simulink model "BESS_F_V_Controle"  (R2017b)
settings: Solver=ode45  StartTime=0.0  StopTime=10  RelTol=1e-3  EnableMultiTasking=on
values from neighbouring files (symbols this model uses):
  beta = beta (k)    [Parameter_2M_DFIG_BESS.m]
  Cbus = 80e-3    (= 0.08)    [Parameter_2M_DFIG_BESS.m]
  Cbus_bess = 15e-3    (= 0.015)    [Parameter_2M_DFIG_BESS.m]
  Cfilter = 80e-3    (= 0.08)    [Parameter_2M_DFIG_BESS.m]
  cp_opt_abs = abs(max(Cp))    [Parameter_2M_DFIG_BESS.m]
  D = 0.1    [Parameter_2M_DFIG_BESS.m]
  f = 60    [Parameter_2M_DFIG_BESS.m]
  Fs = 1.8    [Parameter_2M_DFIG_BESS.m]
  fsw = 4e3    (= 4000)    [Parameter_2M_DFIG_BESS.m]
  J = 90    [Parameter_2M_DFIG_BESS.m]
  ki_id = (wni^2)*Lr*sigma    (= 491.599501999)    [Parameter_2M_DFIG_BESS.m]
  ki_idg = (wnig^2)*Lg    (= 68.6450725305)    [Parameter_2M_DFIG_BESS.m]
  ki_iq = ki_id    (= 491.599501999)    [Parameter_2M_DFIG_BESS.m]
  ki_iqg = ki_idg    (= 68.6450725305)    [Parameter_2M_DFIG_BESS.m]
  ki_v = -300000    [Parameter_2M_DFIG_BESS.m]
  kp_id = (2*wni*sigma*Lr)-Rr    (= 0.5771)    [Parameter_2M_DFIG_BESS.m]
  kp_idg = (2*wnig*Lg)-Rg    (= 0.364153420404)    [Parameter_2M_DFIG_BESS.m]
  kp_iq = kp_id    (= 0.5771)    [Parameter_2M_DFIG_BESS.m]
  kp_iqg = kp_idg    (= 0.364153420404)    [Parameter_2M_DFIG_BESS.m]
  kp_v = -1000    [Parameter_2M_DFIG_BESS.m]
  Kpg = 1/(1.5*Vs*sqrt(2/3))    [Parameter_2M_DFIG_BESS.m]
  Kqg = -Kpg    [Parameter_2M_DFIG_BESS.m]
  lambda_opt = abs(lambda(posicion))    [Parameter_2M_DFIG_BESS.m]
  Lfilter = 483e-6    (= 0.000483)    [Parameter_2M_DFIG_BESS.m]
  Lg = 483e-6    (= 0.000483)    [Parameter_2M_DFIG_BESS.m]
  Lm = 2.5e-3    (= 0.0025)    [Parameter_2M_DFIG_BESS.m]
  Lr = Lm + Lsr    (= 0.002587)    [Parameter_2M_DFIG_BESS.m]
  Ls = Lm + Lsi    (= 0.002587)    [Parameter_2M_DFIG_BESS.m]
  Lsi = 87e-6    (= 8.7e-05)    [Parameter_2M_DFIG_BESS.m]
  N = 100    [Parameter_2M_DFIG_BESS.m]
  p = 2    [Parameter_2M_DFIG_BESS.m]
  Ps = 2e6    (= 2000000)    [Parameter_2M_DFIG_BESS.m]
  Radio = 44    [Parameter_2M_DFIG_BESS.m]
  Rfilter = 20e-3    (= 0.02)    [Parameter_2M_DFIG_BESS.m]
  Rg = 20e-6    (= 2e-05)    [Parameter_2M_DFIG_BESS.m]
  ro = 1.225    [Parameter_2M_DFIG_BESS.m]
  Rr = 2.9e-3    (= 0.0029)    [Parameter_2M_DFIG_BESS.m]
  Rs = 2.6e-3    (= 0.0026)    [Parameter_2M_DFIG_BESS.m]
  sigma = 1- Lm^2/(Ls*Lr)    (= 0.0661284179513)    [Parameter_2M_DFIG_BESS.m]
  Ts = 1/fsw/f    (= 4.16666666667e-06)    [Parameter_2M_DFIG_BESS.m]
  Vbus_ref = 1200    [Parameter_2M_DFIG_BESS.m]
  Vs = 690    [Parameter_2M_DFIG_BESS.m]
undefined symbols (not defined in the file or in its folder): D1, D11, Delta, DiscIntNeverNeededParam, Ion, Lithium, sigbuilder_block
libraries: powerlib x72, powerlib_meascontrol x37, electricdrivelib x1, simulink x1, sps_avr x1
(part 3 of 3)

== system BESS_F_V_Controle/BESS 1.0 MW 690 V/Control System/PI Iq1 ==
  Q*_ref : Inport
  Q_means : Inport  Port=2
  Discrete-Time Integrator : DiscreteIntegrator  SampleTime=1/fsw  LimitOutput=on  UpperSaturationLimit=1e6  LowerSaturationLimit=-Vbus_ref/sqrt(3)  ICPrevOutput=DiscIntNeverNeededParam  ICPrevScaledInput=DiscIntNeverNeededParam
  Error : Display
  Gain : Gain  Gain=kp_iqg
  Gain1 : Gain  Gain=ki_iqg
  Mean : Display
  Mux : Mux  Inputs=3
  Ref : Display
  Sat : Display
  Sat 1 : Display
  Saturation : Saturate  UpperLimit=1e6  LowerLimit=-1e6
  Scope : Scope
  Sum : Sum  Inputs=|+-
  Sum1 : Sum  Inputs=|++
  "Q " : Outport
  wires:
  Sum1/1 -> Saturation/1
  Discrete-Time Integrator/1 -> Sat 1/1, Sum1/2
  Gain1/1 -> Discrete-Time Integrator/1
  Gain/1 -> Sum1/1
  Saturation/1 -> Sat/1, "Q "/1
  Q_means/1 -> Sum/2, Mean/1, Mux/2
  Q*_ref/1 -> Sum/1, Ref/1, Mux/1
  Sum/1 -> Mux/3, Error/1, Gain/1, Gain1/1
  Mux/1 -> Scope/1

== system BESS_F_V_Controle/BESS 1.0 MW 690 V/Control System/PI Iq3 ==
  Vq*_ref : Inport
  Vq_means : Inport  Port=2
  Discrete-Time Integrator : DiscreteIntegrator  SampleTime=1/fsw  LimitOutput=on  UpperSaturationLimit=1e6  LowerSaturationLimit=-1e6  ICPrevOutput=DiscIntNeverNeededParam  ICPrevScaledInput=DiscIntNeverNeededParam
  Error : Display
  Gain4 : Gain  Gain=kp_iq
  Gain5 : Gain  Gain=ki_iq
  Mean : Display
  Mux : Mux  Inputs=3
  Ref : Display
  Sat : Display
  Sat 1 : Display
  Saturation : Saturate  UpperLimit=1e6  LowerLimit=-1e6
  Scope : Scope
  Sum : Sum  Inputs=|+-
  Sum1 : Sum  Inputs=|++
  "Iq " : Outport
  wires:
  Sum1/1 -> Saturation/1
  Discrete-Time Integrator/1 -> Sat 1/1, Sum1/2
  Gain5/1 -> Discrete-Time Integrator/1
  Gain4/1 -> Sum1/1
  Saturation/1 -> Sat/1, "Iq "/1
  Vq_means/1 -> Sum/2, Mean/1, Mux/2
  Vq*_ref/1 -> Sum/1, Ref/1, Mux/1
  Mux/1 -> Scope/1
  Sum/1 -> Gain5/1, Gain4/1, Mux/3, Error/1

== system BESS_F_V_Controle/BESS 1.0 MW 690 V/Control System/PI Iq4 ==
  Vd*_ref : Inport
  Vd_means : Inport  Port=2
  Discrete-Time Integrator : DiscreteIntegrator  SampleTime=1/fsw  LimitOutput=on  UpperSaturationLimit=1e6  LowerSaturationLimit=-1e6  ICPrevOutput=DiscIntNeverNeededParam  ICPrevScaledInput=DiscIntNeverNeededParam
  Error : Display
  Gain4 : Gain  Gain=kp_id
  Gain5 : Gain  Gain=ki_id
  Mean : Display
  Mux : Mux  Inputs=3
  Ref : Display
  Sat : Display
  Sat 1 : Display
  Saturation : Saturate  UpperLimit=1e6  LowerLimit=-1e6
  Scope : Scope
  Sum : Sum  Inputs=|+-
  Sum1 : Sum  Inputs=|++
  "Id " : Outport
  wires:
  Sum1/1 -> Saturation/1
  Discrete-Time Integrator/1 -> Sat 1/1, Sum1/2
  Gain5/1 -> Discrete-Time Integrator/1
  Gain4/1 -> Sum1/1
  Saturation/1 -> Sat/1, "Id "/1
  Vd_means/1 -> Sum/2, Mean/1, Mux/2
  Vd*_ref/1 -> Sum/1, Ref/1, Mux/1
  Sum/1 -> Gain5/1, Gain4/1, Mux/3, Error/1
  Mux/1 -> Scope/1

== system BESS_F_V_Controle/BESS 1.0 MW 690 V/Control System/Q Control ==
  Q*_ref : Inport
  Q_means : Inport  Port=2
  Discrete-Time Integrator : DiscreteIntegrator  SampleTime=1/fsw  LimitOutput=on  UpperSaturationLimit=1.5e6  LowerSaturationLimit=-1.5e6  ICPrevOutput=DiscIntNeverNeededParam  ICPrevScaledInput=DiscIntNeverNeededParam
  Error : Display
  Gain1 : Gain  Gain=kp_idg
  Gain4 : Gain  Gain=ki_idg
  Gain5 : Gain  Gain=Kqg
  Mean : Display
  Mux : Mux  Inputs=3
  Ref : Display
  Sat : Display
  Sat 1 : Display
  Sat1 : Display
  Saturation : Saturate  UpperLimit=1.5e6  LowerLimit=-1.5e6
  Scope : Scope
  Sum : Sum  Inputs=|+-
  Sum1 : Sum  Inputs=|++
  "Q " : Outport
  wires:
  Mux/1 -> Scope/1
  Sum/1 -> Gain4/1, Gain1/1, Error/1, Mux/3
  Q*_ref/1 -> Mux/1, Ref/1, Sum/1
  Q_means/1 -> Mux/2, Mean/1, Sum/2
  Gain1/1 -> Sat1/1, Sum1/1
  Gain4/1 -> Discrete-Time Integrator/1
  Discrete-Time Integrator/1 -> Sum1/2, Sat 1/1
  Sum1/1 -> Saturation/1
  Gain5/1 -> "Q "/1
  Saturation/1 -> Gain5/1, Sat/1

== system BESS_F_V_Controle/BESS 1.0 MW 690 V/Control System/V* ==
  Vd* : Inport
  Vq* : Inport  Port=2
  Display28 : Display
  Fcn : Fcn  Expr=sqrt((u[1])^2-(u[2])^2)
  Mux1 : Mux  Inputs=2
  "V* " : Outport
  wires:
  Vq*/1 -> Mux1/2
  Vd*/1 -> Mux1/1
  Mux1/1 -> Fcn/1
  Fcn/1 -> "V* "/1, Display28/1

== system BESS_F_V_Controle/BESS 1.0 MW 690 V/Control System/Vbus Control ==
  note: signal
  note: reference
  "ref Vbus " : Inport
  "means Vbus " : Inport  Port=2
  Discrete-Time Integrator1 : DiscreteIntegrator  SampleTime=1/fsw  LimitOutput=on  UpperSaturationLimit=0.5e6  LowerSaturationLimit=-0.5e6  ICPrevOutput=DiscIntNeverNeededParam  ICPrevScaledInput=DiscIntNeverNeededParam
  Error : Display
  Gain2 : Gain  Gain=-1000
  Gain3 : Gain  Gain=-300000
  Mean : Display
  Mux : Mux  Inputs=3
  Ref : Display
  Sat : Display
  Sat 1 : Display
  Saturation1 : Saturate  UpperLimit=0.4e6  LowerLimit=-0.4e6
  Scope : Scope
  Sum2 : Sum  Inputs=|+-
  Sum3 : Sum  Inputs=|++
  P_SOC_ref : Outport
  wires:
  Discrete-Time Integrator1/1 -> Sat 1/1, Sum3/2
  Gain3/1 -> Discrete-Time Integrator1/1
  Sum3/1 -> Saturation1/1
  Gain2/1 -> Sum3/1
  Saturation1/1 -> Sat/1, P_SOC_ref/1
  "means Vbus "/1 -> Sum2/2, Mean/1, Mux/2
  "ref Vbus "/1 -> Sum2/1, Ref/1, Mux/1
  Sum2/1 -> Gain2/1, Gain3/1, Mux/3, Error/1
  Mux/1 -> Scope/1

== system BESS_F_V_Controle/BESS 1.0 MW 690 V/Control System/Vmean ==
  Vd* : Inport
  Vq* : Inport  Port=2
  Display28 : Display
  Fcn : Fcn  Expr=sqrt((u[1])^2-(u[2])^2)
  Mux1 : Mux  Inputs=2
  "V* " : Outport
  wires:
  Fcn/1 -> Display28/1, "V* "/1
  Mux1/1 -> Fcn/1
  Vd*/1 -> Mux1/1
  Vq*/1 -> Mux1/2

== system BESS_F_V_Controle/BESS 1.0 MW 690 V/Control System/abc - α//β   ==
  note: iβ_bat
  note: iα_bat
  iabc_bat : Inport
  Fcn : Fcn  Expr=2/3*(u[1]-u[2]/2-u[3]/2)
  Fcn1 : Fcn  Expr=2/3*(u[2]*(sqrt(3)/2)-u[3]*(sqrt(3)/2))
  Mux : Mux  Inputs=2
  i α/β_bat : Outport
  wires:
  Mux/1 -> i α/β_bat/1
  iabc_bat/1 -> Fcn1/1, Fcn/1
  Fcn/1 -> Mux/1
  Fcn1/1 -> Mux/2

== system BESS_F_V_Controle/BESS 1.0 MW 690 V/Control System/abc - α//β  1 ==
  note: iα_bat
  note: iβ_bat
  Vabc_bat : Inport
  Fcn : Fcn  Expr=2/3*(u[1]-u[2]/2-u[3]/2)
  Fcn1 : Fcn  Expr=2/3*(u[2]*(sqrt(3)/2)-u[3]*(sqrt(3)/2))
  Mux : Mux  Inputs=2
  V α/β_bat : Outport
  wires:
  Fcn1/1 -> Mux/2
  Fcn/1 -> Mux/1
  Vabc_bat/1 -> Fcn/1, Fcn1/1
  Mux/1 -> V α/β_bat/1

== system BESS_F_V_Controle/BESS 1.0 MW 690 V/Control System/abc - α//β  2 ==
  note: iβ_bat
  note: iα_bat
  iabc_bat : Inport
  Fcn : Fcn  Expr=2/3*(u[1]-u[2]/2-u[3]/2)
  Fcn1 : Fcn  Expr=2/3*(u[2]*(sqrt(3)/2)-u[3]*(sqrt(3)/2))
  Mux : Mux  Inputs=2
  i α/β_bat : Outport
  wires:
  Mux/1 -> i α/β_bat/1
  iabc_bat/1 -> Fcn1/1, Fcn/1
  Fcn/1 -> Mux/1
  Fcn1/1 -> Mux/2

== system BESS_F_V_Controle/BESS 1.0 MW 690 V/Control System/abc - α//β  3 ==
  note: iα_bat
  note: iβ_bat
  Vabc_bat : Inport
  Fcn : Fcn  Expr=2/3*(u[1]-u[2]/2-u[3]/2)
  Fcn1 : Fcn  Expr=2/3*(u[2]*(sqrt(3)/2)-u[3]*(sqrt(3)/2))
  Mux : Mux  Inputs=2
  V α/β_bat : Outport
  wires:
  Fcn1/1 -> Mux/2
  Fcn/1 -> Mux/1
  Vabc_bat/1 -> Fcn/1, Fcn1/1
  Mux/1 -> V α/β_bat/1

== system BESS_F_V_Controle/BESS 1.0 MW 690 V/Control System/d//q  α//β  ==
  Vdq_bat : Inport
  theta_bat (θ_bat) : Inport  Port=2
  Fcn : Fcn  Expr=u(1)*cos(u[3])-u[2]*sin(u[3])
  Fcn1 : Fcn  Expr=u(1)*sin(u[3])+u[2]*cos(u[3])
  Mux : Mux  Inputs=2
  Mux1 : Mux  Inputs=2
  "Vα/β_bat " : Outport
  wires:
  Mux/1 -> "Vα/β_bat "/1
  Fcn/1 -> Mux/1
  Fcn1/1 -> Mux/2
  Vdq_bat/1 -> Mux1/1
  theta_bat (θ_bat)/1 -> Mux1/2
  Mux1/1 -> Fcn/1, Fcn1/1

== system BESS_F_V_Controle/BESS 1.0 MW 690 V/Control System/α//β - abc ==
  V α/β_bat : Inport
  Fcn : Fcn  Expr=u(1)
  Fcn1 : Fcn  Expr=-(u[1]/2)+u[2]*(sqrt(3)/2)
  Fcn2 : Fcn  Expr=-(u[1]/2)-u[2]*(sqrt(3)/2)
  Mux : Mux  Inputs=3
  Vabc_bat : Outport
  wires:
  Mux/1 -> Vabc_bat/1
  V α/β_bat/1 -> Fcn2/1, Fcn1/1, Fcn/1
  Fcn/1 -> Mux/1
  Fcn1/1 -> Mux/2
  Fcn2/1 -> Mux/3

== system BESS_F_V_Controle/BESS 1.0 MW 690 V/Control System/α//β - d//q ==
  i α/β_bat : Inport
  theta_bat (θ_bat) : Inport  Port=2
  Fcn : Fcn  Expr=u(1)*cos(u[3])+u[2]*sin(u[3])
  Fcn1 : Fcn  Expr=-u(1)*sin(u[3])+u[2]*cos(u[3])
  Mux : Mux  Inputs=2
  Mux1 : Mux  Inputs=2
  i d/q_bat : Outport
  wires:
  Mux/1 -> i d/q_bat/1
  Fcn/1 -> Mux/1
  Fcn1/1 -> Mux/2
  i α/β_bat/1 -> Mux1/1
  theta_bat (θ_bat)/1 -> Mux1/2
  Mux1/1 -> Fcn1/1, Fcn/1

== system BESS_F_V_Controle/BESS 1.0 MW 690 V/Control System/α//β - d//q1 ==
  V α/β_bat : Inport
  theta_bat (θ_bat) : Inport  Port=2
  Fcn : Fcn  Expr=u(1)*cos(u[3])+u[2]*sin(u[3])
  Fcn1 : Fcn  Expr=-u(1)*sin(u[3])+u[2]*cos(u[3])
  Mux : Mux  Inputs=2
  Mux1 : Mux  Inputs=2
  V d/q_bat : Outport
  wires:
  Mux1/1 -> Fcn/1, Fcn1/1
  theta_bat (θ_bat)/1 -> Mux1/2
  V α/β_bat/1 -> Mux1/1
  Fcn1/1 -> Mux/2
  Fcn/1 -> Mux/1
  Mux/1 -> V d/q_bat/1

== system BESS_F_V_Controle/BESS 1.0 MW 690 V/Control System/α//β - d//q2 ==
  i α/β_bat : Inport
  theta_bat (θ_bat) : Inport  Port=2
  Fcn : Fcn  Expr=u(1)*cos(u[3])+u[2]*sin(u[3])
  Fcn1 : Fcn  Expr=-u(1)*sin(u[3])+u[2]*cos(u[3])
  Mux : Mux  Inputs=2
  Mux1 : Mux  Inputs=2
  i d/q_bat : Outport
  wires:
  Mux/1 -> i d/q_bat/1
  Fcn/1 -> Mux/1
  Fcn1/1 -> Mux/2
  i α/β_bat/1 -> Mux1/1
  theta_bat (θ_bat)/1 -> Mux1/2
  Mux1/1 -> Fcn1/1, Fcn/1

== system BESS_F_V_Controle/BESS 1.0 MW 690 V/Control System/α//β - d//q3 ==
  V α/β_bat : Inport
  theta_bat (θ_bat) : Inport  Port=2
  Fcn : Fcn  Expr=u(1)*cos(u[3])+u[2]*sin(u[3])
  Fcn1 : Fcn  Expr=-u(1)*sin(u[3])+u[2]*cos(u[3])
  Mux : Mux  Inputs=2
  Mux1 : Mux  Inputs=2
  V d/q_bat : Outport
  wires:
  Mux1/1 -> Fcn/1, Fcn1/1
  theta_bat (θ_bat)/1 -> Mux1/2
  V α/β_bat/1 -> Mux1/1
  Fcn1/1 -> Mux/2
  Fcn/1 -> Mux/1
  Mux/1 -> V d/q_bat/1

== system BESS_F_V_Controle/DFIG 2.0 MW 690 V1/Control/ Angle Rotor ==
  note: Theta_m (θm)
      | Electric
  note: theta_V θv
  note: The stator reference frame (α - β) is a stationary
      | reference frame.
  note: The relation between the mechanical angle of the shaft and the
      | electrical angle depends on the pole pairs of the machine:
      |
      | θm (electrical) = Pole * θm (mechanical)
  note: theta_s (θs)
  note: Vαs/βs
  note: θs=θv-90°
  note: θs=θr+θm
      | θr=θs-θm
  note: Vector control of the DFIM is performed in a synchronously rotating dq frame, in which the d-axis is aligned, in this case, with the stator flux space vector
  Theta_m (θm) Mechanic : Inport
  Vabcs : Inport  Port=2
  "Clarke: abc - αβ " : Subsystem
  Constant : Constant  Value=pi/2
  Demux : Demux  Outputs=2
  Manual Switch1 : ManualSwitch  CurrentSetting=0
  PLL (3ph)1 : powerlib_meascontrol/PLL/PLL (3ph)  Commented=on  Fmin=45  Par_Init=[0, 60]  ParK=[180, 3200, 1]  TcD=1e-4  MaxRateChangeFreq=12  FilterCutOffFreq=25  Ts=0  AGC=on
      link override Model/abc to dq0: Alignment=Aligned with phase A axis
  Pole Pairs : Gain  Gain=p
  Sum : Sum  Inputs=|+-
  Sum1 : Sum  Inputs=|+-
  θv=tan^(-1) (Vβ/Vα) : Trigonometry  Operator=atan2
  theta_r (θr) : Outport
  wires:
  Vabcs/1 -> PLL (3ph)1/1, "Clarke: abc - αβ "/1(Vabc)
  Demux/2 -> θv=tan^(-1) (Vβ/Vα)/1
  Demux/1 -> θv=tan^(-1) (Vβ/Vα)/2
  "Clarke: abc - αβ "/1("Vαs/βs ") -> Demux/1
  Constant/1 -> Sum/2
  Theta_m (θm) Mechanic/1 -> Pole Pairs/1
  Sum/1 -> Sum1/1
  Sum1/1 -> theta_r (θr)/1
  Pole Pairs/1 -> Sum1/2
  Manual Switch1/1 -> Sum/1
  θv=tan^(-1) (Vβ/Vα)/1 -> Manual Switch1/2
  PLL (3ph)1/2 -> Manual Switch1/1

== system BESS_F_V_Controle/DFIG 2.0 MW 690 V1/Control/3er Harmonic Inyection ==
  in : Inport
  Gain : Gain  Gain=-0.5
  MinMax : MinMax
  MinMax1 : MinMax  Function=max
  Scope : Scope
  Sum : Sum  Inputs=|++
  Sum1 : Sum  Inputs=|++
  out : Outport
  wires:
  in/1 -> Sum1/1, MinMax1/1, MinMax/1
  MinMax/1 -> Sum/1
  MinMax1/1 -> Sum/2
  Sum1/1 -> out/1
  Sum/1 -> Gain/1
  Gain/1 -> Scope/1, Sum1/2

== system BESS_F_V_Controle/DFIG 2.0 MW 690 V1/Control/Cancelation of cc ==
  note: Stator Flux
  note: Ωm rd/s
      | Mechanic
  note: ωs (Hz)
  note: Pole Pairs
  note: ωr = ωs - ωm
  note: ωs (rd/s)
  note: ωm (rd/s)
      | Electrical
  Vd : Inport
  Vq : Inport  Port=2
  omega_m (Ωm) : Inport  Port=3
  Constant : Constant  Value=f
  Constant1 : Constant  Value=Fs
  Fcn : Fcn  Expr=u[1]-u[5]*sigma*Lr*u[4]
  Fcn1 : Fcn  Expr=u[2]+u[5]*sigma*Lr*u[3]+u[5]*(Lm/Ls)*u[6]
  Gain : Gain  Gain=p
  Gain1 : Gain  Gain=2*pi
  Mux : Mux  Inputs=2
  Mux1 : Mux  Inputs=6
  Sum : Sum  Inputs=|+-
  Vdr  Vqr : Outport
  tag scope: omega_s=global, vdr=global, vqr=global
  wires:
  Mux/1 -> Vdr  Vqr/1
  Fcn/1 -> [vdr], Mux/1
  Fcn1/1 -> [vqr], Mux/2
  Vd/1 -> Mux1/1
  Vq/1 -> Mux1/2
  Mux1/1 -> Fcn1/1, Fcn/1
  [idr] -> Mux1/3
  [iqr] -> Mux1/4
  Constant1/1 -> Mux1/6
  omega_m (Ωm)/1 -> Gain/1
  Gain/1 -> Sum/2
  Constant/1 -> Gain1/1
  Gain1/1 -> [omega_s], Sum/1
  Sum/1 -> Mux1/5

== system BESS_F_V_Controle/DFIG 2.0 MW 690 V1/Control/PI Id ==
  idr_ref : Inport
  idr_means : Inport  Port=2
  Discrete-Time Integrator : DiscreteIntegrator  SampleTime=1/fsw  LimitOutput=on  UpperSaturationLimit=Vbus_ref/sqrt(3)  LowerSaturationLimit=-Vbus_ref/sqrt(3)  ICPrevOutput=DiscIntNeverNeededParam  ICPrevScaledInput=DiscIntNeverNeededParam
  Error : Display
  Gain : Gain  Gain=kp_id
  Gain1 : Gain  Gain=ki_id
  Mean : Display
  Mux : Mux  Inputs=3
  Ref : Display
  Sat : Display
  Sat2 : Display
  Saturation : Saturate  UpperLimit=Vbus_ref/sqrt(3)  LowerLimit=-Vbus_ref/sqrt(3)
  Scope : Scope
  Sum : Sum  Inputs=|+-
  Sum1 : Sum  Inputs=|++
  Vd : Outport
  wires:
  idr_means/1 -> Mean/1, Mux/2, Sum/2
  idr_ref/1 -> Ref/1, Mux/1, Sum/1
  Sum/1 -> Gain/1, Gain1/1, Mux/3, Error/1
  Gain/1 -> Sum1/1
  Gain1/1 -> Discrete-Time Integrator/1
  Discrete-Time Integrator/1 -> Sat2/1, Sum1/2
  Sum1/1 -> Saturation/1
  Saturation/1 -> Sat/1, Vd/1
  Mux/1 -> Scope/1

== system BESS_F_V_Controle/DFIG 2.0 MW 690 V1/Control/PI Iq ==
  iqr_ref : Inport
  iqr_means : Inport  Port=2
  Discrete-Time Integrator : DiscreteIntegrator  SampleTime=1/fsw  LimitOutput=on  UpperSaturationLimit=Vbus_ref/sqrt(3)  LowerSaturationLimit=-Vbus_ref/sqrt(3)  ICPrevOutput=DiscIntNeverNeededParam  ICPrevScaledInput=DiscIntNeverNeededParam
  Display1 : Display
  Error : Display
  Gain : Gain  Gain=kp_iq
  Gain1 : Gain  Gain=ki_iq
  Mean : Display
  Mux : Mux  Inputs=3
  Ref : Display
  Sat : Display
  Saturation : Saturate  UpperLimit=Vbus_ref/sqrt(3)  LowerLimit=-Vbus_ref/sqrt(3)
  Scope : Scope
  Sum : Sum  Inputs=|+-
  Sum1 : Sum  Inputs=|++
  Vq : Outport
  wires:
  Gain/1 -> Sum1/1
  Gain1/1 -> Discrete-Time Integrator/1
  Sum1/1 -> Saturation/1
  Discrete-Time Integrator/1 -> Display1/1, Sum1/2
  iqr_means/1 -> Sum/2, Mean/1, Mux/2
  iqr_ref/1 -> Sum/1, Ref/1, Mux/1
  Sum/1 -> Gain/1, Gain1/1, Mux/3, Error/1
  Saturation/1 -> Sat/1, Vq/1
  Mux/1 -> Scope/1

== system BESS_F_V_Controle/DFIG 2.0 MW 690 V1/Control/abc - α//β  ==
  note: iβr
  note: iαr
  iabcr : Inport
  Fcn : Fcn  Expr=2/3*(u[1]-u[2]/2-u[3]/2)
  Fcn1 : Fcn  Expr=2/3*(u[2]*(sqrt(3)/2)-u[3]*(sqrt(3)/2))
  Mux : Mux  Inputs=2
  i αr/βr : Outport
  wires:
  Mux/1 -> i αr/βr/1
  iabcr/1 -> Fcn1/1, Fcn/1
  Fcn/1 -> Mux/1
  Fcn1/1 -> Mux/2

== system BESS_F_V_Controle/DFIG 2.0 MW 690 V1/Control/d//q - α//β ==
  Vdr  Vqr : Inport
  theta_r (θr) : Inport  Port=2
  Fcn : Fcn  Expr=u(1)*cos(u[3])-u[2]*sin(u[3])
  Fcn1 : Fcn  Expr=u(1)*sin(u[3])+u[2]*cos(u[3])
  Mux : Mux  Inputs=2
  Mux1 : Mux  Inputs=2
  V αr/βr : Outport
  wires:
  Mux/1 -> V αr/βr/1
  Fcn/1 -> Mux/1
  Fcn1/1 -> Mux/2
  Vdr  Vqr/1 -> Mux1/1
  theta_r (θr)/1 -> Mux1/2
  Mux1/1 -> Fcn/1, Fcn1/1

== system BESS_F_V_Controle/DFIG 2.0 MW 690 V1/Control/α//β - abc ==
  V αr/βr : Inport
  Fcn : Fcn  Expr=u(1)
  Fcn1 : Fcn  Expr=-(u[1]/2)+u[2]*(sqrt(3)/2)
  Fcn2 : Fcn  Expr=-(u[1]/2)-u[2]*(sqrt(3)/2)
  Mux : Mux  Inputs=3
  Vabcr : Outport
  wires:
  Mux/1 -> Vabcr/1
  V αr/βr/1 -> Fcn2/1, Fcn1/1, Fcn/1
  Fcn/1 -> Mux/1
  Fcn1/1 -> Mux/2
  Fcn2/1 -> Mux/3

== system BESS_F_V_Controle/DFIG 2.0 MW 690 V1/Control/α//β - d//q ==
  i αr/βr : Inport
  theta_r (θr) : Inport  Port=2
  Fcn : Fcn  Expr=u(1)*cos(u[3])+u[2]*sin(u[3])
  Fcn1 : Fcn  Expr=-u(1)*sin(u[3])+u[2]*cos(u[3])
  Mux : Mux  Inputs=2
  Mux1 : Mux  Inputs=2
  i dr/qr : Outport
  wires:
  Mux/1 -> i dr/qr/1
  Fcn/1 -> Mux/1
  Fcn1/1 -> Mux/2
  i αr/βr/1 -> Mux1/1
  theta_r (θr)/1 -> Mux1/2
  Mux1/1 -> Fcn1/1, Fcn/1

== system BESS_F_V_Controle/DFIG 2.0 MW 690 V1/Control1/ Angle Rotor ==
  note: Vg α/β
  "Vabcg " : Inport
  " abc - αβ " : Subsystem
  Demux : Demux  Outputs=2
  θv=tan^(-1) (Vβ/Vα) : Trigonometry  Operator=atan2
  theta_g (θg) : Outport
  wires:
  " abc - αβ "/1("Vg α/β ") -> Demux/1
  Demux/1 -> θv=tan^(-1) (Vβ/Vα)/2
  Demux/2 -> θv=tan^(-1) (Vβ/Vα)/1
  "Vabcg "/1 -> " abc - αβ "/1(Vabcg)
  θv=tan^(-1) (Vβ/Vα)/1 -> theta_g (θg)/1

== system BESS_F_V_Controle/DFIG 2.0 MW 690 V1/Control1/3er Harmonic Inyection ==
  in : Inport
  Gain : Gain  Gain=-0.5
  MinMax : MinMax
  MinMax1 : MinMax  Function=max
  Scope : Scope
  Sum : Sum  Inputs=|++
  Sum1 : Sum  Inputs=|++
  out : Outport
  wires:
  Gain/1 -> Sum1/2, Scope/1
  Sum/1 -> Gain/1
  Sum1/1 -> out/1
  MinMax1/1 -> Sum/2
  MinMax/1 -> Sum/1
  in/1 -> MinMax/1, MinMax1/1, Sum1/1

== system BESS_F_V_Controle/DFIG 2.0 MW 690 V1/Control1/Cancelation of cc ==
  Id : Inport
  Iq : Inport  Port=2
  Display : Display
  Fcn : Fcn  Expr=u[1]-u[4]*Lg*(2*pi*f)
  Fcn1 : Fcn  Expr=u[2]+u[3]*Lg*(2*pi*f)
  Mux : Mux  Inputs=2
  Mux1 : Mux
  Vdg  Vqg : Outport
  tag scope: vdg=global, vqg=global
  wires:
  [iqg] -> Mux1/4
  [idg] -> Mux1/3
  Mux1/1 -> Fcn/1, Fcn1/1
  Iq/1 -> Mux1/2
  Id/1 -> Mux1/1
  Fcn1/1 -> Mux/2, [vqg]
  Fcn/1 -> Mux/1, Display/1, [vdg]
  Mux/1 -> Vdg  Vqg/1

== system BESS_F_V_Controle/DFIG 2.0 MW 690 V1/Control1/PI ==
  note: signal
  note: reference
  "ref Vbus " : Inport
  "means Vbus " : Inport  Port=2
  Discrete-Time Integrator1 : DiscreteIntegrator  SampleTime=1/fsw  LimitOutput=on  UpperSaturationLimit=Ps  LowerSaturationLimit=-Ps  ICPrevOutput=DiscIntNeverNeededParam  ICPrevScaledInput=DiscIntNeverNeededParam
  Error : Display
  Gain2 : Gain  Gain=kp_v
  Gain3 : Gain  Gain=ki_v
  Mean : Display
  Mux : Mux  Inputs=3
  Ref : Display
  Sat : Display
  Sat 1 : Display
  Saturation1 : Saturate  UpperLimit=Ps  LowerLimit=-Ps
  Scope : Scope
  Sum2 : Sum  Inputs=|+-
  Sum3 : Sum  Inputs=|++
  P_rotor_ref : Outport
  wires:
  Discrete-Time Integrator1/1 -> Sat 1/1, Sum3/2
  Gain3/1 -> Discrete-Time Integrator1/1
  Sum3/1 -> Saturation1/1
  Gain2/1 -> Sum3/1
  Saturation1/1 -> Sat/1, P_rotor_ref/1
  "means Vbus "/1 -> Sum2/2, Mean/1, Mux/2
  "ref Vbus "/1 -> Sum2/1, Ref/1, Mux/1
  Sum2/1 -> Gain2/1, Gain3/1, Mux/3, Error/1
  Mux/1 -> Scope/1

== system BESS_F_V_Controle/DFIG 2.0 MW 690 V1/Control1/PI Id ==
  idg_ref : Inport
  idg_means : Inport  Port=2
  Discrete-Time Integrator : DiscreteIntegrator  SampleTime=1/fsw  LimitOutput=on  UpperSaturationLimit=Vbus_ref/sqrt(3)*2  LowerSaturationLimit=-Vbus_ref/sqrt(3)*2  ICPrevOutput=DiscIntNeverNeededParam  ICPrevScaledInput=DiscIntNeverNeededParam
  Error : Display
  Gain : Gain  Gain=kp_idg
  Gain1 : Gain  Gain=ki_idg
  Mean : Display
  Mux : Mux  Inputs=3
  Ref : Display
  Sat : Display
  Sat 1 : Display
  Saturation : Saturate  UpperLimit=Vbus_ref/sqrt(3)*2  LowerLimit=-Vbus_ref/sqrt(3)*2
  Scope : Scope
  Sum : Sum  Inputs=|+-
  Sum1 : Sum  Inputs=|++
  out : Outport
  wires:
  Saturation/1 -> Sat/1, out/1
  Sum1/1 -> Saturation/1
  Discrete-Time Integrator/1 -> Sat 1/1, Sum1/2
  Gain1/1 -> Discrete-Time Integrator/1
  Gain/1 -> Sum1/1
  idg_means/1 -> Mean/1, Mux/2, Sum/2
  idg_ref/1 -> Ref/1, Mux/1, Sum/1
  Sum/1 -> Gain/1, Gain1/1, Mux/3, Error/1
  Mux/1 -> Scope/1

== system BESS_F_V_Controle/DFIG 2.0 MW 690 V1/Control1/PI Iq ==
  iqg_ref : Inport
  iqg_means : Inport  Port=2
  Discrete-Time Integrator : DiscreteIntegrator  SampleTime=1/fsw  LimitOutput=on  UpperSaturationLimit=Vbus_ref/sqrt(3)  LowerSaturationLimit=-Vbus_ref/sqrt(3)  ICPrevOutput=DiscIntNeverNeededParam  ICPrevScaledInput=DiscIntNeverNeededParam
  Error : Display
  Gain : Gain  Gain=kp_iqg
  Gain1 : Gain  Gain=ki_iqg
  Mean : Display
  Mux : Mux  Inputs=3
  Ref : Display
  Sat : Display
  Sat 1 : Display
  Saturation : Saturate  UpperLimit=Vbus_ref/sqrt(3)  LowerLimit=-Vbus_ref/sqrt(3)
  Scope : Scope
  Sum : Sum  Inputs=|+-
  Sum1 : Sum  Inputs=|++
  out : Outport
  wires:
  Sum1/1 -> Saturation/1
  Discrete-Time Integrator/1 -> Sat 1/1, Sum1/2
  Gain1/1 -> Discrete-Time Integrator/1
  Gain/1 -> Sum1/1
  Saturation/1 -> Sat/1, out/1
  iqg_means/1 -> Sum/2, Mean/1, Mux/2
  iqg_ref/1 -> Sum/1, Ref/1, Mux/1
  Sum/1 -> Mux/3, Error/1, Gain/1, Gain1/1
  Mux/1 -> Scope/1

== system BESS_F_V_Controle/DFIG 2.0 MW 690 V1/Control1/abc - α//β   ==
  note: iαg
  note: iβg
  iabcg : Inport
  Fcn : Fcn  Expr=2/3*(u[1]-u[2]/2-u[3]/2)
  Fcn1 : Fcn  Expr=2/3*(u[2]*(sqrt(3)/2)-u[3]*(sqrt(3)/2))
  Mux : Mux  Inputs=2
  i αg/βg : Outport
  wires:
  Fcn1/1 -> Mux/2
  Fcn/1 -> Mux/1
  iabcg/1 -> Fcn/1, Fcn1/1
  Mux/1 -> i αg/βg/1

== system BESS_F_V_Controle/DFIG 2.0 MW 690 V1/Control1/d//q  α//β  ==
  Vdg  Vqg : Inport
  theta_g (θg) : Inport  Port=2
  Fcn : Fcn  Expr=u(1)*cos(u[3])-u[2]*sin(u[3])
  Fcn1 : Fcn  Expr=u(1)*sin(u[3])+u[2]*cos(u[3])
  Mux : Mux  Inputs=2
  Mux1 : Mux  Inputs=2
  V αg/βg : Outport
  wires:
  Mux1/1 -> Fcn1/1, Fcn/1
  theta_g (θg)/1 -> Mux1/2
  Vdg  Vqg/1 -> Mux1/1
  Fcn1/1 -> Mux/2
  Fcn/1 -> Mux/1
  Mux/1 -> V αg/βg/1

== system BESS_F_V_Controle/DFIG 2.0 MW 690 V1/Control1/α//β - abc ==
  V αg/βg : Inport
  Fcn : Fcn  Expr=u(1)
  Fcn1 : Fcn  Expr=-(u[1]/2)+u[2]*(sqrt(3)/2)
  Fcn2 : Fcn  Expr=-(u[1]/2)-u[2]*(sqrt(3)/2)
  Mux : Mux  Inputs=3
  Vabcg : Outport
  wires:
  Fcn2/1 -> Mux/3
  Fcn1/1 -> Mux/2
  Fcn/1 -> Mux/1
  V αg/βg/1 -> Fcn/1, Fcn1/1, Fcn2/1
  Mux/1 -> Vabcg/1

== system BESS_F_V_Controle/DFIG 2.0 MW 690 V1/Control1/α//β - d//q ==
  i αg/βg : Inport
  theta_g (θg) : Inport  Port=2
  Fcn : Fcn  Expr=u(1)*cos(u[3])+u[2]*sin(u[3])
  Fcn1 : Fcn  Expr=-u(1)*sin(u[3])+u[2]*cos(u[3])
  Mux : Mux  Inputs=2
  Mux1 : Mux  Inputs=2
  i dg/qg : Outport
  wires:
  Mux1/1 -> Fcn/1, Fcn1/1
  theta_g (θg)/1 -> Mux1/2
  i αg/βg/1 -> Mux1/1
  Fcn1/1 -> Mux/2
  Fcn/1 -> Mux/1
  Mux/1 -> i dg/qg/1

== system BESS_F_V_Controle/BESS 1.0 MW 690 V/Control System/ Angle Rotor/ abc - αβ  ==
  Vabc_bat : Inport
  Fcn : Fcn  Expr=2/3*(u[1]-u[2]/2-u[3]/2)
  Fcn1 : Fcn  Expr=2/3*(u[2]*(sqrt(3)/2)-u[3]*(sqrt(3)/2))
  Mux : Mux  Inputs=2
  "V α/β_bat " : Outport
  wires:
  Mux/1 -> "V α/β_bat "/1
  Vabc_bat/1 -> Fcn1/1, Fcn/1
  Fcn/1 -> Mux/1
  Fcn1/1 -> Mux/2

== system BESS_F_V_Controle/BESS 1.0 MW 690 V/Control System/ Angle Rotor1/ abc - αβ  ==
  Vabc_bat : Inport
  Fcn : Fcn  Expr=2/3*(u[1]-u[2]/2-u[3]/2)
  Fcn1 : Fcn  Expr=2/3*(u[2]*(sqrt(3)/2)-u[3]*(sqrt(3)/2))
  Mux : Mux  Inputs=2
  "V α/β_bat " : Outport
  wires:
  Mux/1 -> "V α/β_bat "/1
  Vabc_bat/1 -> Fcn1/1, Fcn/1
  Fcn/1 -> Mux/1
  Fcn1/1 -> Mux/2

== system BESS_F_V_Controle/DFIG 2.0 MW 690 V1/Control/ Angle Rotor/Clarke: abc - αβ  ==
  Vabc : Inport
  Fcn : Fcn  Expr=2/3*(u[1]-u[2]/2-u[3]/2)
  Fcn1 : Fcn  Expr=2/3*(u[2]*(sqrt(3)/2)-u[3]*(sqrt(3)/2))
  Mux : Mux  Inputs=2
  "Vαs/βs " : Outport
  wires:
  Mux/1 -> "Vαs/βs "/1
  Vabc/1 -> Fcn1/1, Fcn/1
  Fcn/1 -> Mux/1
  Fcn1/1 -> Mux/2

== system BESS_F_V_Controle/DFIG 2.0 MW 690 V1/Control1/ Angle Rotor/ abc - αβ  ==
  Vabcg : Inport
  Fcn : Fcn  Expr=2/3*(u[1]-u[2]/2-u[3]/2)
  Fcn1 : Fcn  Expr=2/3*(u[2]*(sqrt(3)/2)-u[3]*(sqrt(3)/2))
  Mux : Mux  Inputs=2
  "Vg α/β " : Outport
  wires:
  Fcn1/1 -> Mux/2
  Fcn/1 -> Mux/1
  Vabcg/1 -> Fcn/1, Fcn1/1
  Mux/1 -> "Vg α/β "/1
